simulink model "simple_stateflow1"  (R2024b)
settings: Solver=ode3  StartTime=0.0  StopTime=20.0  FixedStep=1  RelTol=1e-3
libraries: simulink x3
settings Model: Creator=balaj  LastModifiedBy=balaj

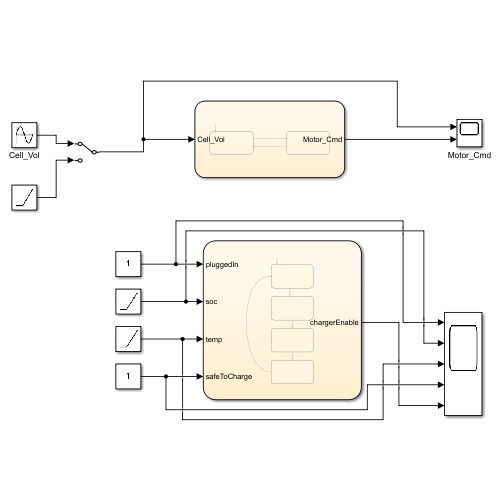
[thumbnail: Simulink's stored preview of the top-level diagram]
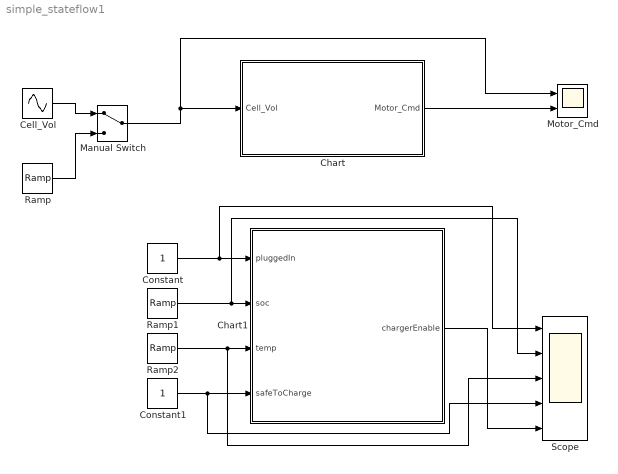
== system simple_stateflow1 ==
  Cell_Vol : Sin  Amplitude=4  SampleTime=0
  Chart : Stateflow chart  TreatAsAtomicUnit=on
  Chart1 : Stateflow chart  TreatAsAtomicUnit=on
  Constant : Constant  OutDataTypeStr=boolean
  Constant1 : Constant  OutDataTypeStr=boolean
  Manual Switch : ManualSwitch
  Motor_Cmd : Scope  NumInputPorts=2
  Ramp : simulink/Sources/Ramp  slope=0.5  start=0  InitialOutput=0
  Ramp1 : simulink/Sources/Ramp  slope=10  start=0  InitialOutput=0
  Ramp2 : simulink/Sources/Ramp  slope=5  start=0  InitialOutput=0
  Scope : Scope  NumInputPorts=5
  wires:
  Chart/1(Motor_Cmd) -> Motor_Cmd/2
  Cell_Vol/1 -> Manual Switch/1
  Ramp/1 -> Manual Switch/2
  Manual Switch/1 -> Motor_Cmd/1, Chart/1(Cell_Vol)
  Constant/1 -> Scope/1, Chart1/1(pluggedIn)
  Ramp1/1 -> Scope/2, Chart1/2(soc)
  Ramp2/1 -> Scope/3, Chart1/3(temp)
  Constant1/1 -> Scope/4, Chart1/4(safeToCharge)
  Chart1/1(chargerEnable) -> Scope/5

== stateflow chart simple_stateflow1/Chart1 ==
  state Idle
    entry:
    chargerEnable=0;
  state PreCharge
    entry:
    chargerEnable=0;
  state Charging
    entry:
    chargerEnable=1;
  state Cutoff
    entry:
    chargerEnable=0;
  (default) -> Idle
  Cutoff -> Idle : [pluggedIn==0]
  Idle -> PreCharge : [pluggedIn==1]
  PreCharge -> Charging : [safeToCharge==1]
  Charging -> Cutoff : [soc>=95 || temp>=45]
  data: pluggedIn input boolean; soc input double; temp input double; safeToCharge input boolean; chargerEnable output

== stateflow chart simple_stateflow1/Chart ==
  state Standby
    entry:
    Motor_Cmd=0;
  state Running
    entry:
    Motor_Cmd=0.5;
  (default) -> Standby
  Standby -> Running : [Cell_Vol>3.6]
  Running -> Standby : [Cell_Vol<=3.6]
  data: Cell_Vol input; Motor_Cmd output
